simulink model "TestStructure"  (R2023b)
settings: Solver=FixedStepDiscrete  StartTime=0.0  StopTime=inf  FixedStep=SampleTime  RelTol=1e-3
InitFcn:
  | SampleTime = 0.001;
  | ButtonValue=0;
  | load("BusConfig.mat");
undefined symbols (not defined in the file): DiscIntNeverNeededParam
libraries: slrealtimeethercatlib x219, dspfdesign x28, dspstat3 x23, simulink x21, slpidlib x10, dspswit3 x8, commfilt2 x2, dspsigops x1
(part 3 of 8)

== system TestStructure/Bus/Subsystem5/Enabled Subsystem ==
  In1 : Inport
  In2 : Inport  Port=2
  Enable : EnablePort
  Set Device State : slrealtimeethercatlib/Set Device State  device_id=0  slave_name=Drive 2 (Elmo Drive )  sample_time=-1  slave_addr=1002  selected_slave=Term 1 (EK1100)  slave_found=1
  Out1 : Outport
  Out2 : Outport  Port=2
  wires:
  In1/1 -> Set Device State/1
  Set Device State/2 -> Out2/1
  In2/1 -> Set Device State/2
  Set Device State/1 -> Out1/1

== system TestStructure/Bus/Subsystem5/Enabled Subsystem1 ==
  In3 : Inport
  Enable : EnablePort
  EtherCAT Async SDO Upload : slrealtimeethercatlib/EtherCAT Async SDO Upload  index=0x6075  subIndex=0  sig_type=uint32  sig_dim=1  device_id=0  slave_name=Drive 2 (Elmo Drive )  sample_time=-1  slave_addr=1002  selected_slave=Term 1 (EK1100)  timeout=3000  slave_found=1  complete=0
  Out3 : Outport
  Out4 : Outport  Port=2
  Out5 : Outport  Port=3
  wires:
  EtherCAT Async SDO Upload/3 -> Out5/1
  In3/1 -> EtherCAT Async SDO Upload/1
  EtherCAT Async SDO Upload/2 -> Out4/1
  EtherCAT Async SDO Upload/1 -> Out3/1

== system TestStructure/Bus/Subsystem5/Enabled Subsystem2 ==
  In4 : Inport
  In5 : Inport  Port=2
  Enable : EnablePort
  EtherCAT Async SDO Download : slrealtimeethercatlib/EtherCAT Async SDO Download  index=0x6080  subIndex=0  sig_type=int32  sig_dim=1  device_id=0  slave_name=Drive 2 (Elmo Drive )  sample_time=-1  slave_addr=1002  selected_slave=Term 1 (EK1100)  timeout=3000  slave_found=1  complete=0
  Out6 : Outport
  Out7 : Outport  Port=2
  wires:
  EtherCAT Async SDO Download/2 -> Out7/1
  In4/1 -> EtherCAT Async SDO Download/1
  In5/1 -> EtherCAT Async SDO Download/2
  EtherCAT Async SDO Download/1 -> Out6/1

== system TestStructure/Bus/Subsystem5/Enabled Subsystem3 ==
  In6 : Inport
  In7 : Inport  Port=2
  Enable : EnablePort
  EtherCAT Async SDO Download1 : slrealtimeethercatlib/EtherCAT Async SDO Download  index=0x6060  subIndex=0  sig_type=int8  sig_dim=1  device_id=0  slave_name=Drive 2 (Elmo Drive )  sample_time=-1  slave_addr=1002  selected_slave=Term 1 (EK1100)  timeout=2000  slave_found=1  complete=0
  Out8 : Outport
  Out9 : Outport  Port=2
  wires:
  In6/1 -> EtherCAT Async SDO Download1/1
  EtherCAT Async SDO Download1/1 -> Out8/1
  In7/1 -> EtherCAT Async SDO Download1/2
  EtherCAT Async SDO Download1/2 -> Out9/1

== system TestStructure/Bus/Subsystem5/Enabled Subsystem4 ==
  In8 : Inport
  In9 : Inport  Port=2
  Enable : EnablePort
  Set Device State1 : slrealtimeethercatlib/Set Device State  device_id=0  slave_name=Drive 2 (Elmo Drive )  sample_time=-1  slave_addr=1002  selected_slave=Term 1 (EK1100)  slave_found=1
  Out10 : Outport
  Out11 : Outport  Port=2
  wires:
  Set Device State1/1 -> Out10/1
  In8/1 -> Set Device State1/1
  In9/1 -> Set Device State1/2
  Set Device State1/2 -> Out11/1

== system TestStructure/Bus/Subsystem5/Enabled Subsystem5 ==
  Enable : EnablePort
  Get Device State : slrealtimeethercatlib/Get Device State  device_id=0  slave_name=Drive 2 (Elmo Drive )  sample_time=0.001  slave_addr=1002  selected_slave=Term 1 (EK1100)  timeout=500  slave_found=1
  Out12 : Outport
  wires:
  Get Device State/1 -> Out12/1

== system TestStructure/Bus/Subsystem5/Enabled Subsystem6 ==
  In10 : Inport
  Enable : EnablePort
  EtherCAT PDO Receive1 : slrealtimeethercatlib/EtherCAT PDO Receive  Priority=2  sig_name=Drive 2 (Elmo Drive ).Inputs.Status word  sig_offset=12544  sig_type=uint16  type_size=16  sig_dim=1  device_id=0  sample_time=0.001000
  EtherCAT PDO Transmit1 : slrealtimeethercatlib/EtherCAT PDO Transmit  Priority=3  sig_name=Drive 2 (Elmo Drive ).Outputs.Control word  sig_offset=12512  sig_type=uint16  type_size=16  sig_dim=1  device_id=0  sample_time=0.001000
  Out13 : Outport
  wires:
  EtherCAT PDO Receive1/1 -> Out13/1
  In10/1 -> EtherCAT PDO Transmit1/1

== system TestStructure/Bus/Subsystem5/Enabled Subsystem7 ==
  Enable : EnablePort
  EtherCAT PDO Receive2 : slrealtimeethercatlib/EtherCAT PDO Receive  Priority=2  sig_name=Drive 2 (Elmo Drive ).Inputs.Position actual value  sig_offset=12496  sig_type=int32  type_size=32  sig_dim=1  device_id=0  sample_time=0.001000
  Out1 : Outport
  wires:
  EtherCAT PDO Receive2/1 -> Out1/1

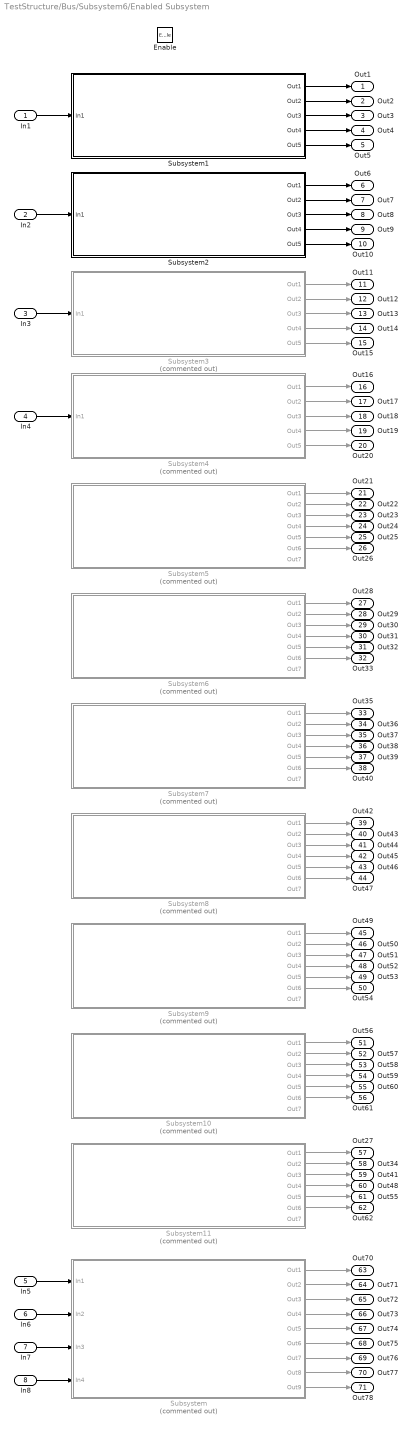
== system TestStructure/Bus/Subsystem6/Enabled Subsystem ==
  In1 : Inport
  In2 : Inport  Port=2
  In3 : Inport  Port=3
  In4 : Inport  Port=4
  In5 : Inport  Port=5
  In6 : Inport  Port=6
  In7 : Inport  Port=7
  In8 : Inport  Port=8
  Enable : EnablePort
  Subsystem : Subsystem  Commented=on
  Subsystem1 : Subsystem
  Subsystem10 : Subsystem  Commented=on
  Subsystem11 : Subsystem  Commented=on
  Subsystem2 : Subsystem
  Subsystem3 : Subsystem  Commented=on
  Subsystem4 : Subsystem  Commented=on
  Subsystem5 : Subsystem  Commented=on
  Subsystem6 : Subsystem  Commented=on
  Subsystem7 : Subsystem  Commented=on
  Subsystem8 : Subsystem  Commented=on
  Subsystem9 : Subsystem  Commented=on
  Out1 : Outport
  Out2 : Outport  Port=2
  Out3 : Outport  Port=3
  Out4 : Outport  Port=4
  Out5 : Outport  Port=5
  Out6 : Outport  Port=6
  Out7 : Outport  Port=7
  Out8 : Outport  Port=8
  Out9 : Outport  Port=9
  Out10 : Outport  Port=10
  Out11 : Outport  Port=11
  Out12 : Outport  Port=12
  Out13 : Outport  Port=13
  Out14 : Outport  Port=14
  Out15 : Outport  Port=15
  Out16 : Outport  Port=16
  Out17 : Outport  Port=17
  Out18 : Outport  Port=18
  Out19 : Outport  Port=19
  Out20 : Outport  Port=20
  Out21 : Outport  Port=21
  Out22 : Outport  Port=22
  Out23 : Outport  Port=23
  Out24 : Outport  Port=24
  Out25 : Outport  Port=25
  Out26 : Outport  Port=26
  Out28 : Outport  Port=27
  Out29 : Outport  Port=28
  Out30 : Outport  Port=29
  Out31 : Outport  Port=30
  Out32 : Outport  Port=31
  Out33 : Outport  Port=32
  Out35 : Outport  Port=33
  Out36 : Outport  Port=34
  Out37 : Outport  Port=35
  Out38 : Outport  Port=36
  Out39 : Outport  Port=37
  Out40 : Outport  Port=38
  Out42 : Outport  Port=39
  Out43 : Outport  Port=40
  Out44 : Outport  Port=41
  Out45 : Outport  Port=42
  Out46 : Outport  Port=43
  Out47 : Outport  Port=44
  Out49 : Outport  Port=45
  Out50 : Outport  Port=46
  Out51 : Outport  Port=47
  Out52 : Outport  Port=48
  Out53 : Outport  Port=49
  Out54 : Outport  Port=50
  Out56 : Outport  Port=51
  Out57 : Outport  Port=52
  Out58 : Outport  Port=53
  Out59 : Outport  Port=54
  Out60 : Outport  Port=55
  Out61 : Outport  Port=56
  Out27 : Outport  Port=57
  Out34 : Outport  Port=58
  Out41 : Outport  Port=59
  Out48 : Outport  Port=60
  Out55 : Outport  Port=61
  Out62 : Outport  Port=62
  Out70 : Outport  Port=63
  Out71 : Outport  Port=64
  Out72 : Outport  Port=65
  Out73 : Outport  Port=66
  Out74 : Outport  Port=67
  Out75 : Outport  Port=68
  Out76 : Outport  Port=69
  Out77 : Outport  Port=70
  Out78 : Outport  Port=71
  wires:
  In1/1 -> Subsystem1/1(In1)
  In2/1 -> Subsystem2/1(In1)
  In3/1 -> Subsystem3/1(In1)
  In4/1 -> Subsystem4/1(In1)
  Subsystem1/1(Out1) -> Out1/1
  Subsystem1/2(Out2) -> Out2/1
  Subsystem1/3(Out3) -> Out3/1
  Subsystem1/4(Out4) -> Out4/1
  Subsystem1/5(Out5) -> Out5/1
  Subsystem2/1(Out1) -> Out6/1
  Subsystem2/2(Out2) -> Out7/1
  Subsystem2/3(Out3) -> Out8/1
  Subsystem2/4(Out4) -> Out9/1
  Subsystem2/5(Out5) -> Out10/1
  Subsystem3/1(Out1) -> Out11/1
  Subsystem3/2(Out2) -> Out12/1
  Subsystem3/3(Out3) -> Out13/1
  Subsystem3/4(Out4) -> Out14/1
  Subsystem3/5(Out5) -> Out15/1
  Subsystem4/1(Out1) -> Out16/1
  Subsystem4/2(Out2) -> Out17/1
  Subsystem4/3(Out3) -> Out18/1
  Subsystem4/4(Out4) -> Out19/1
  Subsystem4/5(Out5) -> Out20/1
  Subsystem5/1(Out1) -> Out21/1
  Subsystem5/2(Out2) -> Out22/1
  Subsystem5/3(Out3) -> Out23/1
  Subsystem5/4(Out4) -> Out24/1
  Subsystem5/5(Out5) -> Out25/1
  Subsystem5/6(Out6) -> Out26/1
  Subsystem6/1(Out1) -> Out28/1
  Subsystem6/2(Out2) -> Out29/1
  Subsystem6/3(Out3) -> Out30/1
  Subsystem6/4(Out4) -> Out31/1
  Subsystem6/5(Out5) -> Out32/1
  Subsystem6/6(Out6) -> Out33/1
  Subsystem7/1(Out1) -> Out35/1
  Subsystem7/2(Out2) -> Out36/1
  Subsystem7/3(Out3) -> Out37/1
  Subsystem7/4(Out4) -> Out38/1
  Subsystem7/5(Out5) -> Out39/1
  Subsystem7/6(Out6) -> Out40/1
  Subsystem8/1(Out1) -> Out42/1
  Subsystem8/2(Out2) -> Out43/1
  Subsystem8/3(Out3) -> Out44/1
  Subsystem8/4(Out4) -> Out45/1
  Subsystem8/5(Out5) -> Out46/1
  Subsystem8/6(Out6) -> Out47/1
  Subsystem9/1(Out1) -> Out49/1
  Subsystem9/2(Out2) -> Out50/1
  Subsystem9/3(Out3) -> Out51/1
  Subsystem9/4(Out4) -> Out52/1
  Subsystem9/5(Out5) -> Out53/1
  Subsystem9/6(Out6) -> Out54/1
  Subsystem10/1(Out1) -> Out56/1
  Subsystem10/2(Out2) -> Out57/1
  Subsystem10/3(Out3) -> Out58/1
  Subsystem10/4(Out4) -> Out59/1
  Subsystem10/5(Out5) -> Out60/1
  Subsystem10/6(Out6) -> Out61/1
  In5/1 -> Subsystem/1(In1)
  In6/1 -> Subsystem/2(In2)
  In7/1 -> Subsystem/3(In3)
  In8/1 -> Subsystem/4(In4)
  Subsystem/1(Out1) -> Out70/1
  Subsystem/2(Out2) -> Out71/1
  Subsystem/3(Out3) -> Out72/1
  Subsystem/4(Out4) -> Out73/1
  Subsystem/5(Out5) -> Out74/1
  Subsystem/6(Out6) -> Out75/1
  Subsystem/7(Out7) -> Out76/1
  Subsystem/8(Out8) -> Out77/1
  Subsystem/9(Out9) -> Out78/1
  Subsystem11/1(Out1) -> Out27/1
  Subsystem11/2(Out2) -> Out34/1
  Subsystem11/3(Out3) -> Out41/1
  Subsystem11/4(Out4) -> Out48/1
  Subsystem11/5(Out5) -> Out55/1
  Subsystem11/6(Out6) -> Out62/1

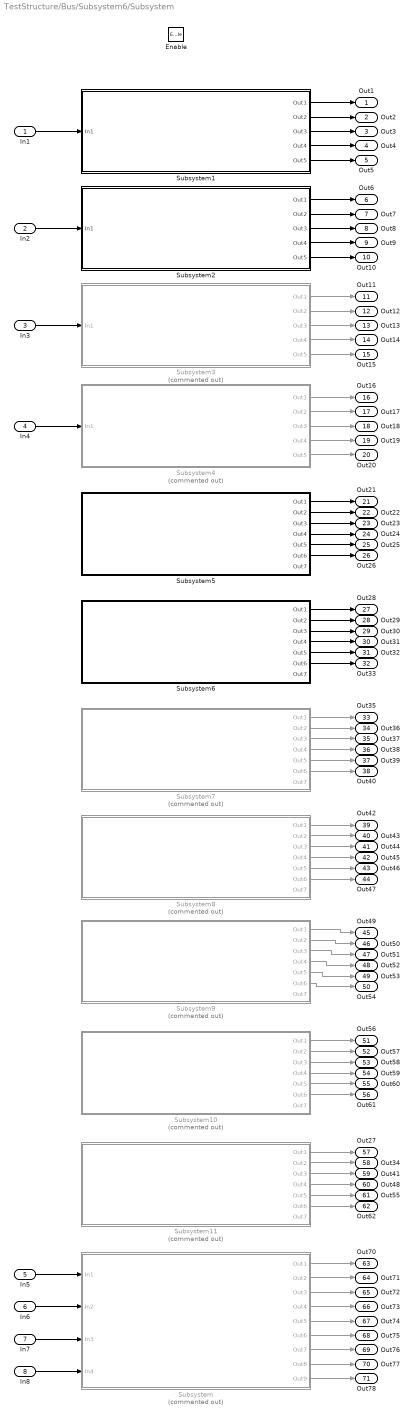
== system TestStructure/Bus/Subsystem6/Subsystem ==
  In1 : Inport
  In2 : Inport  Port=2
  In3 : Inport  Port=3
  In4 : Inport  Port=4
  In5 : Inport  Port=5
  In6 : Inport  Port=6
  In7 : Inport  Port=7
  In8 : Inport  Port=8
  Enable : EnablePort
  Subsystem : Subsystem  Commented=on
  Subsystem1 : Subsystem
  Subsystem10 : Subsystem  Commented=on
  Subsystem11 : Subsystem  Commented=on
  Subsystem2 : Subsystem
  Subsystem3 : Subsystem  Commented=on
  Subsystem4 : Subsystem  Commented=on
  Subsystem5 : Subsystem
  Subsystem6 : Subsystem
  Subsystem7 : Subsystem  Commented=on
  Subsystem8 : Subsystem  Commented=on
  Subsystem9 : Subsystem  Commented=on
  Out1 : Outport
  Out2 : Outport  Port=2
  Out3 : Outport  Port=3
  Out4 : Outport  Port=4
  Out5 : Outport  Port=5
  Out6 : Outport  Port=6
  Out7 : Outport  Port=7
  Out8 : Outport  Port=8
  Out9 : Outport  Port=9
  Out10 : Outport  Port=10
  Out11 : Outport  Port=11
  Out12 : Outport  Port=12
  Out13 : Outport  Port=13
  Out14 : Outport  Port=14
  Out15 : Outport  Port=15
  Out16 : Outport  Port=16
  Out17 : Outport  Port=17
  Out18 : Outport  Port=18
  Out19 : Outport  Port=19
  Out20 : Outport  Port=20
  Out21 : Outport  Port=21
  Out22 : Outport  Port=22
  Out23 : Outport  Port=23
  Out24 : Outport  Port=24
  Out25 : Outport  Port=25
  Out26 : Outport  Port=26
  Out28 : Outport  Port=27
  Out29 : Outport  Port=28
  Out30 : Outport  Port=29
  Out31 : Outport  Port=30
  Out32 : Outport  Port=31
  Out33 : Outport  Port=32
  Out35 : Outport  Port=33
  Out36 : Outport  Port=34
  Out37 : Outport  Port=35
  Out38 : Outport  Port=36
  Out39 : Outport  Port=37
  Out40 : Outport  Port=38
  Out42 : Outport  Port=39
  Out43 : Outport  Port=40
  Out44 : Outport  Port=41
  Out45 : Outport  Port=42
  Out46 : Outport  Port=43
  Out47 : Outport  Port=44
  Out49 : Outport  Port=45
  Out50 : Outport  Port=46
  Out51 : Outport  Port=47
  Out52 : Outport  Port=48
  Out53 : Outport  Port=49
  Out54 : Outport  Port=50
  Out56 : Outport  Port=51
  Out57 : Outport  Port=52
  Out58 : Outport  Port=53
  Out59 : Outport  Port=54
  Out60 : Outport  Port=55
  Out61 : Outport  Port=56
  Out27 : Outport  Port=57
  Out34 : Outport  Port=58
  Out41 : Outport  Port=59
  Out48 : Outport  Port=60
  Out55 : Outport  Port=61
  Out62 : Outport  Port=62
  Out70 : Outport  Port=63
  Out71 : Outport  Port=64
  Out72 : Outport  Port=65
  Out73 : Outport  Port=66
  Out74 : Outport  Port=67
  Out75 : Outport  Port=68
  Out76 : Outport  Port=69
  Out77 : Outport  Port=70
  Out78 : Outport  Port=71
  wires:
  Subsystem/7(Out7) -> Out76/1
  Subsystem5/5(Out5) -> Out25/1
  Subsystem/8(Out8) -> Out77/1
  Subsystem/9(Out9) -> Out78/1
  Subsystem5/1(Out1) -> Out21/1
  Subsystem7/4(Out4) -> Out38/1
  Subsystem/6(Out6) -> Out75/1
  Subsystem/5(Out5) -> Out74/1
  Subsystem4/4(Out4) -> Out19/1
  Subsystem1/1(Out1) -> Out1/1
  Subsystem/3(Out3) -> Out72/1
  Subsystem8/6(Out6) -> Out47/1
  Subsystem/4(Out4) -> Out73/1
  Subsystem8/5(Out5) -> Out46/1
  Subsystem6/6(Out6) -> Out33/1
  Subsystem5/3(Out3) -> Out23/1
  Subsystem3/5(Out5) -> Out15/1
  Subsystem4/5(Out5) -> Out20/1
  Subsystem3/3(Out3) -> Out13/1
  Subsystem2/5(Out5) -> Out10/1
  Subsystem4/1(Out1) -> Out16/1
  Subsystem8/1(Out1) -> Out42/1
  Subsystem8/4(Out4) -> Out45/1
  Subsystem4/3(Out3) -> Out18/1
  Subsystem10/4(Out4) -> Out59/1
  Subsystem8/2(Out2) -> Out43/1
  Subsystem/2(Out2) -> Out71/1
  Subsystem10/2(Out2) -> Out57/1
  Subsystem9/6(Out6) -> Out54/1
  Subsystem4/2(Out2) -> Out17/1
  Subsystem7/6(Out6) -> Out40/1
  Subsystem9/2(Out2) -> Out50/1
  Subsystem7/2(Out2) -> Out36/1
  Subsystem7/3(Out3) -> Out37/1
  Subsystem3/4(Out4) -> Out14/1
  Subsystem5/2(Out2) -> Out22/1
  Subsystem10/6(Out6) -> Out61/1
  Subsystem6/3(Out3) -> Out30/1
  Subsystem2/3(Out3) -> Out8/1
  Subsystem/1(Out1) -> Out70/1
  Subsystem2/1(Out1) -> Out6/1
  Subsystem3/1(Out1) -> Out11/1
  Subsystem5/6(Out6) -> Out26/1
  Subsystem7/5(Out5) -> Out39/1
  Subsystem1/3(Out3) -> Out3/1
  Subsystem3/2(Out2) -> Out12/1
  Subsystem9/3(Out3) -> Out51/1
  Subsystem10/1(Out1) -> Out56/1
  Subsystem6/2(Out2) -> Out29/1
  Subsystem2/2(Out2) -> Out7/1
  Subsystem1/5(Out5) -> Out5/1
  Subsystem9/4(Out4) -> Out52/1
  Subsystem1/4(Out4) -> Out4/1
  Subsystem6/4(Out4) -> Out31/1
  Subsystem5/4(Out4) -> Out24/1
  Subsystem10/5(Out5) -> Out60/1
  Subsystem1/2(Out2) -> Out2/1
  Subsystem2/4(Out4) -> Out9/1
  Subsystem9/5(Out5) -> Out53/1
  Subsystem7/1(Out1) -> Out35/1
  Subsystem6/1(Out1) -> Out28/1
  Subsystem8/3(Out3) -> Out44/1
  Subsystem9/1(Out1) -> Out49/1
  Subsystem10/3(Out3) -> Out58/1
  Subsystem6/5(Out5) -> Out32/1
  In3/1 -> Subsystem3/1(In1)
  In5/1 -> Subsystem/1(In1)
  In2/1 -> Subsystem2/1(In1)
  In1/1 -> Subsystem1/1(In1)
  In8/1 -> Subsystem/4(In4)
  In7/1 -> Subsystem/3(In3)
  In4/1 -> Subsystem4/1(In1)
  In6/1 -> Subsystem/2(In2)
  Subsystem11/1(Out1) -> Out27/1
  Subsystem11/2(Out2) -> Out34/1
  Subsystem11/3(Out3) -> Out41/1
  Subsystem11/4(Out4) -> Out48/1
  Subsystem11/5(Out5) -> Out55/1
  Subsystem11/6(Out6) -> Out62/1

== system TestStructure/Bus/Subsystem6/Subsystem2 ==
  Enable : EnablePort
  Subsystem7 : Subsystem
  Subsystem8 : Subsystem
  Out35 : Outport
  Out36 : Outport  Port=2
  Out37 : Outport  Port=3
  Out38 : Outport  Port=4
  Out42 : Outport  Port=5
  Out43 : Outport  Port=6
  Out44 : Outport  Port=7
  Out45 : Outport  Port=8
  wires:
  Subsystem7/1(Out1) -> Out35/1
  Subsystem8/3(Out3) -> Out44/1
  Subsystem7/4(Out4) -> Out38/1
  Subsystem7/3(Out3) -> Out37/1
  Subsystem8/2(Out2) -> Out43/1
  Subsystem7/2(Out2) -> Out36/1
  Subsystem8/1(Out1) -> Out42/1
  Subsystem8/4(Out4) -> Out45/1

== system TestStructure/Bus/Subsystem7/Enabled Subsystem ==
  In1 : Inport
  In2 : Inport  Port=2
  Enable : EnablePort
  Set Device State : slrealtimeethercatlib/Set Device State  device_id=0  slave_name=Drive 2 (Elmo Drive )  sample_time=-1  slave_addr=1002  selected_slave=Term 1 (EK1100)  slave_found=1
  Out1 : Outport
  Out2 : Outport  Port=2
  wires:
  In1/1 -> Set Device State/1
  Set Device State/2 -> Out2/1
  In2/1 -> Set Device State/2
  Set Device State/1 -> Out1/1

== system TestStructure/Bus/Subsystem7/Enabled Subsystem1 ==
  In3 : Inport
  Enable : EnablePort
  EtherCAT Async SDO Upload : slrealtimeethercatlib/EtherCAT Async SDO Upload  index=0x6075  subIndex=0  sig_type=uint32  sig_dim=1  device_id=0  slave_name=Drive 2 (Elmo Drive )  sample_time=-1  slave_addr=1002  selected_slave=Term 1 (EK1100)  timeout=3000  slave_found=1  complete=0
  Out3 : Outport
  Out4 : Outport  Port=2
  Out5 : Outport  Port=3
  wires:
  EtherCAT Async SDO Upload/3 -> Out5/1
  In3/1 -> EtherCAT Async SDO Upload/1
  EtherCAT Async SDO Upload/2 -> Out4/1
  EtherCAT Async SDO Upload/1 -> Out3/1

== system TestStructure/Bus/Subsystem7/Enabled Subsystem2 ==
  In4 : Inport
  In5 : Inport  Port=2
  Enable : EnablePort
  EtherCAT Async SDO Download : slrealtimeethercatlib/EtherCAT Async SDO Download  index=0x6080  subIndex=0  sig_type=int32  sig_dim=1  device_id=0  slave_name=Drive 2 (Elmo Drive )  sample_time=-1  slave_addr=1002  selected_slave=Term 1 (EK1100)  timeout=3000  slave_found=1  complete=0
  Out6 : Outport
  Out7 : Outport  Port=2
  wires:
  EtherCAT Async SDO Download/2 -> Out7/1
  In4/1 -> EtherCAT Async SDO Download/1
  In5/1 -> EtherCAT Async SDO Download/2
  EtherCAT Async SDO Download/1 -> Out6/1

== system TestStructure/Bus/Subsystem7/Enabled Subsystem3 ==
  In6 : Inport
  In7 : Inport  Port=2
  Enable : EnablePort
  EtherCAT Async SDO Download1 : slrealtimeethercatlib/EtherCAT Async SDO Download  index=0x6060  subIndex=0  sig_type=int8  sig_dim=1  device_id=0  slave_name=Drive 2 (Elmo Drive )  sample_time=-1  slave_addr=1002  selected_slave=Term 1 (EK1100)  timeout=2000  slave_found=1  complete=0
  Out8 : Outport
  Out9 : Outport  Port=2
  wires:
  In6/1 -> EtherCAT Async SDO Download1/1
  EtherCAT Async SDO Download1/1 -> Out8/1
  In7/1 -> EtherCAT Async SDO Download1/2
  EtherCAT Async SDO Download1/2 -> Out9/1

== system TestStructure/Bus/Subsystem7/Enabled Subsystem4 ==
  In8 : Inport
  In9 : Inport  Port=2
  Enable : EnablePort
  Set Device State1 : slrealtimeethercatlib/Set Device State  device_id=0  slave_name=Drive 2 (Elmo Drive )  sample_time=-1  slave_addr=1002  selected_slave=Term 1 (EK1100)  slave_found=1
  Out10 : Outport
  Out11 : Outport  Port=2
  wires:
  Set Device State1/1 -> Out10/1
  In8/1 -> Set Device State1/1
  In9/1 -> Set Device State1/2
  Set Device State1/2 -> Out11/1

== system TestStructure/Bus/Subsystem7/Enabled Subsystem5 ==
  Enable : EnablePort
  Get Device State : slrealtimeethercatlib/Get Device State  device_id=0  slave_name=Drive 2 (Elmo Drive )  sample_time=0.001  slave_addr=1002  selected_slave=Term 1 (EK1100)  timeout=500  slave_found=1
  Out12 : Outport
  wires:
  Get Device State/1 -> Out12/1

== system TestStructure/Bus/Subsystem7/Enabled Subsystem6 ==
  In10 : Inport
  Enable : EnablePort
  EtherCAT PDO Receive1 : slrealtimeethercatlib/EtherCAT PDO Receive  Priority=2  sig_name=Drive 2 (Elmo Drive ).Inputs.Status word  sig_offset=12544  sig_type=uint16  type_size=16  sig_dim=1  device_id=0  sample_time=0.001000
  EtherCAT PDO Transmit1 : slrealtimeethercatlib/EtherCAT PDO Transmit  Priority=3  sig_name=Drive 2 (Elmo Drive ).Outputs.Control word  sig_offset=12512  sig_type=uint16  type_size=16  sig_dim=1  device_id=0  sample_time=0.001000
  Out13 : Outport
  wires:
  EtherCAT PDO Receive1/1 -> Out13/1
  In10/1 -> EtherCAT PDO Transmit1/1

== system TestStructure/Bus/Subsystem7/Enabled Subsystem7 ==
  Enable : EnablePort
  EtherCAT PDO Receive2 : slrealtimeethercatlib/EtherCAT PDO Receive  Priority=2  sig_name=Drive 2 (Elmo Drive ).Inputs.Position actual value  sig_offset=12496  sig_type=int32  type_size=32  sig_dim=1  device_id=0  sample_time=0.001000
  Out1 : Outport
  wires:
  EtherCAT PDO Receive2/1 -> Out1/1

== system TestStructure/InterForceControlTask/AO/Filter ==
  In : Inport
  Highpass Filter : dspfdesign/Highpass Filter  FilterType=IIR  DesignForMinimumOrder=on  FilterOrder=50  StopbandFrequency=0.015  PassbandFrequency=0.3  StopbandAttenuation=80  PassbandRipple=0.1  SampleRateMode=Specify on dialog  SampleRate=1000  SimulateUsing=Interpreted execution  roundingMode=Floor  coeffsDataTypeStr=fixdt(1,16)
  Highpass Filter1 : dspfdesign/Highpass Filter  FilterType=IIR  DesignForMinimumOrder=on  FilterOrder=50  StopbandFrequency=0.29  PassbandFrequency=0.3  StopbandAttenuation=60  PassbandRipple=1  SampleRateMode=Specify on dialog  SampleRate=1000  SimulateUsing=Code generation  roundingMode=Floor  coeffsDataTypeStr=fixdt(1,16)
  Lowpass Filter : dspfdesign/Lowpass Filter  FilterType=IIR  DesignForMinimumOrder=on  FilterOrder=50  PassbandFrequency=2.3  StopbandFrequency=4.3  PassbandRipple=0.1  StopbandAttenuation=80  SampleRateMode=Specify on dialog  SampleRate=1000  SimulateUsing=Interpreted execution  roundingMode=Floor  coeffsDataTypeStr=fixdt(1,16)
  Lowpass Filter1 : dspfdesign/Lowpass Filter  FilterType=IIR  DesignForMinimumOrder=on  FilterOrder=50  PassbandFrequency=6  StopbandFrequency=8  PassbandRipple=1  StopbandAttenuation=60  SampleRateMode=Specify on dialog  SampleRate=1000  SimulateUsing=Code generation  roundingMode=Floor  coeffsDataTypeStr=fixdt(1,16)
  Out : Outport
  wires:
  Highpass Filter1/1 -> Lowpass Filter1/1
  In/1 -> Highpass Filter1/1
  Lowpass Filter1/1 -> Out/1
  Highpass Filter/1 -> Lowpass Filter/1

== system TestStructure/InterForceControlTask/AO/PhaseCorrection ==
  note: Subsystem
  Peaks : Inport
  T_base_default : Inport  Port=2
  Clock : Clock
  Constant3 : Constant
  Discrete-Time Integrator : DiscreteIntegrator  ExternalReset=rising  SampleTime=-1  ICPrevOutput=DiscIntNeverNeededParam  ICPrevScaledInput=DiscIntNeverNeededParam
  If : If  IfExpression=u1 == 1
  If Action Subsystem : Subsystem  TreatAsAtomicUnit=on
  If Action Subsystem1 : Subsystem  TreatAsAtomicUnit=on
  MATLAB Function : MATLAB Function  TreatAsAtomicUnit=on
  MATLAB Function1 : MATLAB Function  TreatAsAtomicUnit=on
  MATLAB Function2 : MATLAB Function  TreatAsAtomicUnit=on
  Merge : Merge
  Omega : Outport  OutputWhenDisabled=reset  InitialOutput=[0]
  Phi_Corrected : Outport  Port=2  OutputWhenDisabled=reset  InitialOutput=[0]
  wires:
  Clock/1 -> MATLAB Function1/2(t)
  Peaks/1 -> MATLAB Function2/1(valid_peak), If/1, MATLAB Function1/1(raw_peak)
  If/1 -> If Action Subsystem/Action
  Discrete-Time Integrator/1 -> MATLAB Function/1(t_t_start)
  If/2 -> If Action Subsystem1/Action
  Merge/1 -> Discrete-Time Integrator/2, MATLAB Function/2(u)
  Constant3/1 -> Discrete-Time Integrator/1
  If Action Subsystem1/1(Out1) -> Merge/2
  If Action Subsystem/1(Out1) -> Merge/1
  MATLAB Function/1(Omega) -> Omega/1
  MATLAB Function/2(phi) -> Phi_Corrected/1
  T_base_default/1 -> MATLAB Function/3(T_base_default)

== system TestStructure/InterForceControlTask/AO/Select ==
  P : Inport
  Phi : Inport  Port=2
  q : Inport  Port=3
  Abs : Abs  SaturateOnIntegerOverflow=off
  Add : Sum
  Bias1 : Bias  SaturateOnIntegerOverflow=off
  Bias2 : Bias  Bias=-0.001  SaturateOnIntegerOverflow=off
  Constant1 : Constant
  Data Type Conversion : DataTypeConversion  OutDataTypeStr=double  SaturateOnIntegerOverflow=off  RndMeth=Floor
  Edge Detector : dspswit3/Edge Detector
  Gain1 : Gain  Gain=0.6
  Gain2 : Gain  OutDataTypeStr=Inherit: Same as input  ParamDataTypeStr=Inherit: Same as input
  Gain3 : Gain  Gain=0.4
  If Action Subsystem : Subsystem  TreatAsAtomicUnit=on
  If Action Subsystem1 : Subsystem  TreatAsAtomicUnit=on
  If1 : If  NumInputs=3  IfExpression=(u1 >= 10.5)|(u2 <= u3)
  MATLAB Function1 : MATLAB Function  TreatAsAtomicUnit=on
  MO_AOActivityMovment : Sum
  MO_AOActivityThreadhold : Constant  Value=0
  Merge : Merge
  Merge1 : Merge
  Merge2 : Merge
  Moving Average : dspstat3/Moving Average  Method=Sliding window  ForgettingFactorPort=off  SpecifyWindowLength=on  WindowLength=2000  OverlapLength=1999  AllowArbitraryInputLength=off  ForgettingFactor=0.9  SimulateUsing=Code generation
  Moving Average1 : dspstat3/Moving Average  Method=Sliding window  ForgettingFactorPort=off  SpecifyWindowLength=on  WindowLength=2000  OverlapLength=1999  AllowArbitraryInputLength=off  ForgettingFactor=0.9  SimulateUsing=Code generation
  Saturation : Saturate  UpperLimit=inf  LowerLimit=0
  Phi_Out : Outport
  Phase0Event : Outport  Port=2
  PhaseEn : Outport  Port=3
  wires:
  Merge2/1 -> PhaseEn/1
  If Action Subsystem/3(En) -> Merge2/2
  If Action Subsystem1/3(Out3) -> Merge2/1
  Constant1/1 -> If1/1
  Bias1/1 -> If Action Subsystem/2(Phase0)
  If Action Subsystem/2(Phase0Event) -> Merge1/2
  If Action Subsystem1/2(Out2) -> Merge1/1
  If Action Subsystem/1(Phi_Out) -> Merge/2
  MO_AOActivityMovment/1 -> If1/2
  Data Type Conversion/1 -> Gain2/1
  Gain3/1 -> MO_AOActivityMovment/1
  Moving Average1/1 -> MO_AOActivityMovment/2
  q/1 -> MATLAB Function1/1(u)
  MATLAB Function1/1(y) -> Abs/1
  Abs/1 -> Moving Average1/1, Gain3/1
  Merge1/1 -> Phase0Event/1
  Merge/1 -> Phi_Out/1
  If1/2 -> If Action Subsystem/Action
  Add/1 -> ?
  If1/1 -> If Action Subsystem1/Action
  Gain2/1 -> Bias1/1
  Moving Average/1 -> Add/2
  Saturation/1 -> Edge Detector/1
  Edge Detector/1 -> Data Type Conversion/1
  Phi/1 -> If Action Subsystem/1(Phi), Bias2/1
  Bias2/1 -> Saturation/1
  P/1 -> Moving Average/1, Gain1/1
  Gain1/1 -> Add/1
  If Action Subsystem1/1(Out1) -> Merge/1
  MO_AOActivityThreadhold/1 -> If1/3

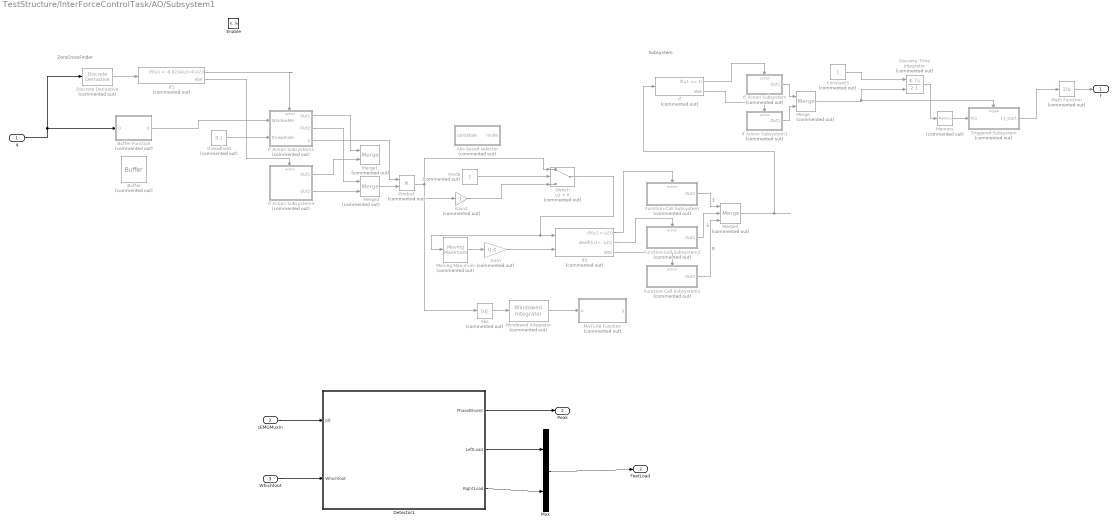
== system TestStructure/InterForceControlTask/AO/Subsystem1 ==
  note: ZeroCrossFinder
  note: Subsystem
  q : Inport
  sEMGMuxIn : Inport  Port=2
  Whichfoot : Inport  Port=3
  Enable : EnablePort  StatesWhenEnabling=reset
  Abs : Abs  Commented=on  SaturateOnIntegerOverflow=off
  Abs-based selector : Subsystem  Commented=on
  Buffer : Buffer  Commented=on  N=30  V=29  OutputFrames=off
  Buffer Function : MATLAB Function  Commented=on  TreatAsAtomicUnit=on
  Constant3 : Constant  Commented=on
  Detector1 : Subsystem
  Discrete Derivative : simulink/Discrete/Discrete Derivative  Commented=on  gainval=1.0  ICPrevScaledInput=0.0  OutMin=[]  OutMax=[]  OutDataType=fixdt(1, 16)  OutScaling=2^-10  DoSatur=off
  Discrete-Time Integrator : DiscreteIntegrator  Commented=on  ExternalReset=rising  SampleTime=-1  ICPrevOutput=DiscIntNeverNeededParam  ICPrevScaledInput=DiscIntNeverNeededParam
  Function-Call Subsystem : Subsystem  Commented=on  TreatAsAtomicUnit=on
  Function-Call Subsystem1 : Subsystem  Commented=on  TreatAsAtomicUnit=on
  Function-Call Subsystem2 : Subsystem  Commented=on  TreatAsAtomicUnit=on
  Gain : Gain  Commented=on  Gain=0.4
  Gain2 : Gain  Commented=on  Gain=-1
  If : If  Commented=on  IfExpression=u1 == 1
  If Action Subsystem : Subsystem  Commented=on  TreatAsAtomicUnit=on
  If Action Subsystem1 : Subsystem  Commented=on  TreatAsAtomicUnit=on
  If Action Subsystem2 : Subsystem  Commented=on  TreatAsAtomicUnit=on
  If Action Subsystem3 : Subsystem  Commented=on  TreatAsAtomicUnit=on
  If1 : If  Commented=on  IfExpression=(u1 > -0.02)&(u1<0.02)
  If2 : If  Commented=on  NumInputs=2  IfExpression=(u1 > u2)  ElseIfExpressions=(u1< -u2)
  MATLAB Function : MATLAB Function  Commented=on  TreatAsAtomicUnit=on
  Math Function : Math  Commented=on  Operator=reciprocal
  Memory : Memory  Commented=on
  Merge : Merge  Commented=on
  Merge1 : Merge  Commented=on
  Merge2 : Merge  Commented=on
  Merge3 : Merge  Commented=on  Inputs=3
  Moving Maximum : dspstat3/Moving Maximum  Commented=on  SpecifyWindowLength=on  WindowLength=2000  SimulateUsing=Code generation
  Mux : Mux  Inputs=2
  Product : Product  Commented=on
  Switch : Switch  Commented=on  Criteria=u2 > Threshold  SaturateOnIntegerOverflow=off  InputSameDT=off
  Triggered Subsystem : Subsystem  Commented=on  TreatAsAtomicUnit=on
  Windowed Integrator : commfilt2/Windowed Integrator  Commented=on  integperiod=600  roundingMode=Floor  overflowMode=off  coeffDataTypeStr=Inherit: Same word length as input  coeffMin=[]  coeffMax=[]  coeffLastDataTypeStr=Inherit: Same word length as input  accumDataTypeStr=Inherit: Same as product output  accumLastDataTypeStr=Inherit: Same as product output  outputDataTypeStr=Inherit: Same as accumulator  outputMin=[]  outputMax=[]  outputLastDataTypeStr=Inherit: Same as accumulator
  mode : Constant  Commented=on
  threadhold : Constant  Commented=on  Value=0.1
  f : Outport
  Peak : Outport  Port=2  OutputWhenDisabled=reset  InitialOutput=[0]
  FeetLoad : Outport  Port=3  OutputWhenDisabled=reset  InitialOutput=[0]
  wires:
  Triggered Subsystem/1(t-t_start) -> Math Function/1
  Math Function/1 -> f/1
  Memory/1 -> Triggered Subsystem/1(In1)
  If Action Subsystem/1(Out1) -> Merge/1
  If Action Subsystem1/1(Out1) -> Merge/2
  Constant3/1 -> Discrete-Time Integrator/1
  If/1 -> If Action Subsystem/Action
  Merge/1 -> Discrete-Time Integrator/2, Triggered Subsystem/Trigger
  If/2 -> If Action Subsystem1/Action
  Discrete-Time Integrator/1 -> Memory/1
  q/1 -> Discrete Derivative/1, Buffer Function/1(u)
  If Action Subsystem3/1(Out1) -> Merge1/2
  If Action Subsystem2/1(Out1) -> Merge1/1
  If1/2 -> If Action Subsystem3/Action
  If1/1 -> If Action Subsystem2/Action
  Discrete Derivative/1 -> If1/1
  Buffer Function/1(y) -> If Action Subsystem2/1(WindowMin)
  If Action Subsystem2/2(Out2) -> Merge2/1
  If Action Subsystem3/2(Out2) -> Merge2/2
  Merge2/1 -> Product/2
  If Action Subsystem2/3(y) -> Product/1
  Function-Call Subsystem/1(Out1) -> Merge3/1  "1"
  Function-Call Subsystem1/1(Out1) -> Merge3/3  "0"
  If2/1 -> Function-Call Subsystem/Action
  If2/3 -> Function-Call Subsystem1/Action
  Function-Call Subsystem2/1(Out1) -> Merge3/2  "-1"
  If2/2 -> Function-Call Subsystem2/Action
  Moving Maximum/1 -> Gain/1
  Gain/1 -> If2/2
  Product/1 -> Switch/1, Abs/1, Gain2/1
  Switch/1 -> Moving Maximum/1, If2/1
  Gain2/1 -> Switch/3
  threadhold/1 -> If Action Subsystem2/2(threadhold)
  Abs/1 -> Windowed Integrator/1
  Windowed Integrator/1 -> MATLAB Function/1(u)
  mode/1 -> Switch/2
  Merge3/1 -> If/1
  Detector1/1(Phase0Event) -> Peak/1
  sEMGMuxIn/1 -> Detector1/1(p8)
  Whichfoot/1 -> Detector1/2(Whichfoot)
  Detector1/2(LeftLoad) -> Mux/1
  Detector1/3(RightLoad) -> Mux/2
  Mux/1 -> FeetLoad/1

== system TestStructure/InterForceControlTask/AO1/Filter ==
  In : Inport
  Highpass Filter : dspfdesign/Highpass Filter  FilterType=IIR  DesignForMinimumOrder=on  FilterOrder=50  StopbandFrequency=0.015  PassbandFrequency=0.3  StopbandAttenuation=80  PassbandRipple=0.1  SampleRateMode=Specify on dialog  SampleRate=1000  SimulateUsing=Interpreted execution  roundingMode=Floor  coeffsDataTypeStr=fixdt(1,16)
  Highpass Filter1 : dspfdesign/Highpass Filter  FilterType=IIR  DesignForMinimumOrder=on  FilterOrder=50  StopbandFrequency=0.2  PassbandFrequency=0.3  StopbandAttenuation=60  PassbandRipple=1  SampleRateMode=Specify on dialog  SampleRate=1000  SimulateUsing=Code generation  roundingMode=Floor  coeffsDataTypeStr=fixdt(1,16)
  Lowpass Filter : dspfdesign/Lowpass Filter  FilterType=IIR  DesignForMinimumOrder=on  FilterOrder=50  PassbandFrequency=2.3  StopbandFrequency=4.3  PassbandRipple=0.1  StopbandAttenuation=80  SampleRateMode=Specify on dialog  SampleRate=1000  SimulateUsing=Interpreted execution  roundingMode=Floor  coeffsDataTypeStr=fixdt(1,16)
  Lowpass Filter1 : dspfdesign/Lowpass Filter  FilterType=IIR  DesignForMinimumOrder=on  FilterOrder=50  PassbandFrequency=6  StopbandFrequency=8  PassbandRipple=1  StopbandAttenuation=60  SampleRateMode=Specify on dialog  SampleRate=1000  SimulateUsing=Code generation  roundingMode=Floor  coeffsDataTypeStr=fixdt(1,16)
  Out : Outport
  wires:
  Highpass Filter1/1 -> Lowpass Filter1/1
  In/1 -> Highpass Filter/1
  Lowpass Filter/1 -> Out/1
  Highpass Filter/1 -> Lowpass Filter/1

== system TestStructure/InterForceControlTask/AO1/PhaseCorrection ==
  note: Subsystem
  Peaks : Inport
  Clock : Clock
  Constant3 : Constant
  Discrete-Time Integrator : DiscreteIntegrator  ExternalReset=rising  SampleTime=-1  ICPrevOutput=DiscIntNeverNeededParam  ICPrevScaledInput=DiscIntNeverNeededParam
  If : If  IfExpression=u1 == 1
  If Action Subsystem : Subsystem  TreatAsAtomicUnit=on
  If Action Subsystem1 : Subsystem  TreatAsAtomicUnit=on
  MATLAB Function : MATLAB Function  TreatAsAtomicUnit=on
  MATLAB Function1 : MATLAB Function  TreatAsAtomicUnit=on
  MATLAB Function2 : MATLAB Function  TreatAsAtomicUnit=on
  Merge : Merge
  Omega : Outport  OutputWhenDisabled=reset  InitialOutput=[0]
  Phi_Corrected : Outport  Port=2  OutputWhenDisabled=reset  InitialOutput=[0]
  wires:
  Clock/1 -> MATLAB Function1/2(t)
  MATLAB Function1/1(valid_peak) -> If/1, MATLAB Function2/1(valid_peak)
  Peaks/1 -> MATLAB Function1/1(raw_peak)
  If/1 -> If Action Subsystem/Action
  Discrete-Time Integrator/1 -> MATLAB Function/1(t_t_start)
  If/2 -> If Action Subsystem1/Action
  Merge/1 -> Discrete-Time Integrator/2, MATLAB Function/2(u)
  Constant3/1 -> Discrete-Time Integrator/1
  If Action Subsystem1/1(Out1) -> Merge/2
  If Action Subsystem/1(Out1) -> Merge/1
  MATLAB Function/1(Omega) -> Omega/1
  MATLAB Function/2(phi) -> Phi_Corrected/1

== system TestStructure/InterForceControlTask/AO1/Select ==
  P : Inport
  Phi : Inport  Port=2
  q : Inport  Port=3
  Abs : Abs  SaturateOnIntegerOverflow=off
  Add : Sum
  Add1 : Sum
  Bias1 : Bias  SaturateOnIntegerOverflow=off
  Bias2 : Bias  Bias=-0.001  SaturateOnIntegerOverflow=off
  Constant1 : Constant
  Data Type Conversion : DataTypeConversion  OutDataTypeStr=double  SaturateOnIntegerOverflow=off  RndMeth=Floor
  Edge Detector : dspswit3/Edge Detector
  Gain1 : Gain  Gain=0.6
  Gain2 : Gain  OutDataTypeStr=Inherit: Same as input  ParamDataTypeStr=Inherit: Same as input
  Gain3 : Gain  Gain=0.6
  If : If  NumInputs=2  IfExpression=(u1 >= 10.5)|(u2 <= 1.5)
  If Action Subsystem : Subsystem  TreatAsAtomicUnit=on
  If Action Subsystem1 : Subsystem  TreatAsAtomicUnit=on
  MATLAB Function1 : MATLAB Function  TreatAsAtomicUnit=on
  Merge : Merge
  Merge1 : Merge
  Merge2 : Merge
  Moving Average : dspstat3/Moving Average  Method=Sliding window  ForgettingFactorPort=off  SpecifyWindowLength=on  WindowLength=2000  OverlapLength=1999  AllowArbitraryInputLength=off  ForgettingFactor=0.9  SimulateUsing=Code generation
  Moving Average1 : dspstat3/Moving Average  Method=Sliding window  ForgettingFactorPort=off  SpecifyWindowLength=on  WindowLength=2000  OverlapLength=1999  AllowArbitraryInputLength=off  ForgettingFactor=0.9  SimulateUsing=Code generation
  Saturation : Saturate  UpperLimit=inf  LowerLimit=0
  Phi_Out : Outport
  Phase0Event : Outport  Port=2
  PhaseEn : Outport  Port=3
  wires:
  Merge2/1 -> PhaseEn/1
  If Action Subsystem/3(En) -> Merge2/2
  If Action Subsystem1/3(Out3) -> Merge2/1
  Constant1/1 -> If/1
  Bias1/1 -> If Action Subsystem/2(Phase0)
  If Action Subsystem/2(Phase0Event) -> Merge1/2
  If Action Subsystem1/2(Out2) -> Merge1/1
  If Action Subsystem/1(Phi_Out) -> Merge/2
  Add1/1 -> If/2
  Data Type Conversion/1 -> Gain2/1
  Gain3/1 -> Add1/1
  Moving Average1/1 -> Add1/2
  q/1 -> MATLAB Function1/1(u)
  MATLAB Function1/1(y) -> Abs/1
  Abs/1 -> Moving Average1/1, Gain3/1
  Merge1/1 -> Phase0Event/1
  Merge/1 -> Phi_Out/1
  If/2 -> If Action Subsystem/Action
  Add/1 -> ?
  If/1 -> If Action Subsystem1/Action
  Gain2/1 -> Bias1/1
  Moving Average/1 -> Add/2
  Saturation/1 -> Edge Detector/1
  Edge Detector/1 -> Data Type Conversion/1
  Phi/1 -> If Action Subsystem/1(Phi), Bias2/1
  Bias2/1 -> Saturation/1
  P/1 -> Moving Average/1, Gain1/1
  Gain1/1 -> Add/1
  If Action Subsystem1/1(Out1) -> Merge/1

== system TestStructure/InterForceControlTask/AO1/Subsystem ==
  q : Inport
  f : Inport  Port=2
  Add : Sum  Inputs=++++
  Gain1 : Gain  Gain=1/(2*pi)
  Gain2 : Gain  Gain=1/(2*pi)
  Subsystem : Subsystem
      settings: PortSchema="{\"entries\":[{\"content\":{\"sides\":[{\"content\":{\"connectorIds\":[\"In1\",\"In2\",\"In3\"]},\"type\":\"ConnectorPlacement.EquallySpacedRectSide\",\"uuid\":\"fcadf485-1c54-4f3f-872d-ec2f9b882f19\"},{\"content\":{\"connectorIds\":[\"Out1\",\"Out2\",\"Out3\",\"Out4\"],\"side\":\"RIGHT\"},\"type\":\"ConnectorPlacement.EquallySpacedRectSide\",\"uuid\":\"c1591880-cfe2-422f-a22e-44609bf238b6\"},{\"content\":{\"connectorIds\":[\"In4\"],\"side\":\"TOP\"},\"type\":\"ConnectorPlacement.EquallySpacedRectSide\",\"uuid\":\"5e5eda86-5041-4cab-91db-6a7c0e12be81\"}]},\"type\":\"ConnectorPlacement.EquallySpacedConnector\",\"uuid\":\"19c16159-ed31-430a-9428-452ee8c26aba\"}],\"packageUris\":[\"http://schema.mathworks.com/mf0/Connector/R2020b\"],\"version\":\"1.0\"}"
  Subsystem1 : Subsystem
  Subsystem2 : Subsystem
      settings: PortSchema="{\"entries\":[{\"content\":{\"sides\":[{\"content\":{\"connectorIds\":[\"In1\",\"In2\",\"In3\"]},\"type\":\"ConnectorPlacement.EquallySpacedRectSide\",\"uuid\":\"8ec379b7-ae46-4480-a29c-58696021cca5\"},{\"content\":{\"connectorIds\":[\"Out1\",\"Out2\",\"Out3\"],\"side\":\"RIGHT\"},\"type\":\"ConnectorPlacement.EquallySpacedRectSide\",\"uuid\":\"cda231b2-17f5-4d36-92f5-7ce39ba724b7\"},{\"content\":{\"connectorIds\":[],\"side\":\"TOP\"},\"type\":\"ConnectorPlacement.EquallySpacedRectSide\",\"uuid\":\"4db6421b-b56f-479d-b059-30db4d04c79c\"},{\"content\":{\"connectorIds\":[\"Out4\"],\"side\":\"BOTTOM\"},\"type\":\"ConnectorPlacement.EquallySpacedRectSide\",\"uuid\":\"ff0451e3-8881-4680-9eeb-8c81f572143a\"}]},\"type\":\"ConnectorPlacement.EquallySpacedConnector\",\"uuid\":\"26cfb436-360b-4c37-a6b2-80fa044f0317\"}],\"packageUris\":[\"http://schema.mathworks.com/mf0/Connector/R2020b\"],\"version\":\"1.0\"}"
  Subsystem3 : Subsystem
  Subsystem5 : Subsystem
  x : Outport
  Omega : Outport  Port=2
  Phi : Outport  Port=3
  P : Outport  Port=4
  wires:
  f/1 -> Subsystem/4(f)
  Subsystem/2(Omega) -> Subsystem1/3(Omega), Subsystem3/2(Omega), Subsystem5/3(Omega), Gain1/1
  Subsystem2/4(P) -> P/1
  Subsystem5/1(x) -> Add/4
  Subsystem3/1(x) -> Add/3
  Subsystem2/3(P(t)_Phi) -> Subsystem/3(P(t)_Phi), Subsystem1/2(P(t)_Phi), Subsystem3/3(P(t)_Phi), Subsystem5/2(P(t)_Phi)
  Subsystem1/1(x) -> Add/2
  Subsystem2/2(P(t)_Omega) -> Subsystem/2(P(t)_Omega)
  Subsystem2/1(P(t)_x) -> Subsystem/1(P(t)_x), Subsystem1/1(P(t)_x), Subsystem3/1(P(t)_x), Subsystem5/1(P(t)_x)
  Gain1/1 -> Omega/1
  Subsystem/3(Phi) -> Gain2/1
  Subsystem/1(x) -> Add/1
  Gain2/1 -> Phi/1
  Add/1 -> x/1, Subsystem2/2(X(t))
  q/1 -> Subsystem2/1(T(t))

== system TestStructure/InterForceControlTask/AO1/Subsystem1 ==
  note: Subsystem
  note: ZeroCrossFinder
  q : Inport
  Enable : EnablePort  StatesWhenEnabling=reset
  Constant3 : Constant
  Discrete Derivative : simulink/Discrete/Discrete Derivative  gainval=1.0  ICPrevScaledInput=0.0  OutMin=[]  OutMax=[]  OutDataType=fixdt(1, 16)  OutScaling=2^-10  DoSatur=off
  Discrete-Time Integrator : DiscreteIntegrator  ExternalReset=rising  SampleTime=-1  ICPrevOutput=DiscIntNeverNeededParam  ICPrevScaledInput=DiscIntNeverNeededParam
  If : If  IfExpression=u1 == 1
  If Action Subsystem : Subsystem  TreatAsAtomicUnit=on
  If Action Subsystem1 : Subsystem  TreatAsAtomicUnit=on
  If Action Subsystem2 : Subsystem  TreatAsAtomicUnit=on
  If Action Subsystem3 : Subsystem  TreatAsAtomicUnit=on
  If1 : If  IfExpression=(u1 > -0.005)|(u1<0.005)
  Math Function : Math  Operator=reciprocal
  Memory : Memory
  Merge : Merge
  Merge1 : Merge
  Moving Minimum : dspstat3/Moving Minimum  SpecifyWindowLength=on  WindowLength=3  SimulateUsing=Code generation
  Triggered Subsystem : Subsystem  TreatAsAtomicUnit=on
  f : Outport
  Peak : Outport  Port=2  OutputWhenDisabled=reset  InitialOutput=[0]
  wires:
  Discrete Derivative/1 -> If1/1
  If1/1 -> If Action Subsystem2/Action
  If1/2 -> If Action Subsystem3/Action
  If Action Subsystem2/1(Out1) -> Merge1/1
  If Action Subsystem3/1(Out1) -> Merge1/2
  q/1 -> Discrete Derivative/1, Moving Minimum/1
  Moving Minimum/1 -> If Action Subsystem2/1(WindowMin)
  Discrete-Time Integrator/1 -> Memory/1
  Merge1/1 -> Peak/1, If/1
  If/2 -> If Action Subsystem1/Action
  Merge/1 -> Triggered Subsystem/Trigger, Discrete-Time Integrator/2
  If/1 -> If Action Subsystem/Action
  Constant3/1 -> Discrete-Time Integrator/1
  If Action Subsystem1/1(Out1) -> Merge/2
  If Action Subsystem/1(Out1) -> Merge/1
  Memory/1 -> Triggered Subsystem/1(In1)
  Math Function/1 -> f/1
  Triggered Subsystem/1(t-t_start) -> Math Function/1

== system TestStructure/InterForceControlTask/AO2/Filter ==
  In : Inport
  Highpass Filter : dspfdesign/Highpass Filter  FilterType=IIR  DesignForMinimumOrder=on  FilterOrder=50  StopbandFrequency=0.015  PassbandFrequency=0.3  StopbandAttenuation=80  PassbandRipple=0.1  SampleRateMode=Specify on dialog  SampleRate=1000  SimulateUsing=Interpreted execution  roundingMode=Floor  coeffsDataTypeStr=fixdt(1,16)
  Highpass Filter1 : dspfdesign/Highpass Filter  Commented=on  FilterType=IIR  DesignForMinimumOrder=on  FilterOrder=50  StopbandFrequency=0.2  PassbandFrequency=0.3  StopbandAttenuation=60  PassbandRipple=1  SampleRateMode=Specify on dialog  SampleRate=1000  SimulateUsing=Code generation  roundingMode=Floor  coeffsDataTypeStr=fixdt(1,16)
  Lowpass Filter : dspfdesign/Lowpass Filter  FilterType=IIR  DesignForMinimumOrder=on  FilterOrder=50  PassbandFrequency=2.3  StopbandFrequency=4.3  PassbandRipple=0.1  StopbandAttenuation=80  SampleRateMode=Specify on dialog  SampleRate=1000  SimulateUsing=Interpreted execution  roundingMode=Floor  coeffsDataTypeStr=fixdt(1,16)
  Lowpass Filter1 : dspfdesign/Lowpass Filter  Commented=on  FilterType=IIR  DesignForMinimumOrder=on  FilterOrder=50  PassbandFrequency=6  StopbandFrequency=8  PassbandRipple=1  StopbandAttenuation=60  SampleRateMode=Specify on dialog  SampleRate=1000  SimulateUsing=Code generation  roundingMode=Floor  coeffsDataTypeStr=fixdt(1,16)
  Out : Outport
  wires:
  Highpass Filter1/1 -> Lowpass Filter1/1
  In/1 -> Highpass Filter/1
  Lowpass Filter/1 -> Out/1
  Highpass Filter/1 -> Lowpass Filter/1

== system TestStructure/InterForceControlTask/AO2/PhaseCorrection ==
  Peaks : Inport
  Phi_GP : Inport  Port=2
  Omega : Inport  Port=3
  Reset : Inport  Port=4
  Constant : Constant  Value=0
  Discrete-Time Integrator : DiscreteIntegrator  ExternalReset=falling  InitialConditionSource=external  SampleTime=-1  ICPrevOutput=DiscIntNeverNeededParam  ICPrevScaledInput=DiscIntNeverNeededParam
  Gain : Gain  Gain=-1
  Math Function : Math
  Product : Product  Inputs=4
  Product1 : Product
  Subsystem : Subsystem
  Subsystem1 : Subsystem
  Subsystem2 : Subsystem
  Subsystem3 : Subsystem
  Subsystem4 : Subsystem
  Subsystem5 : Subsystem
  Subtract : Sum  Inputs=+-
  Phi_Corrected : Outport
  wires:
  Subsystem4/1(k_e) -> Product/1
  Constant/1 -> Discrete-Time Integrator/3
  Subsystem5/1(Phi_Corrected) -> Phi_Corrected/1
  Reset/1 -> Subsystem4/1(Reset), Discrete-Time Integrator/2
  Math Function/1 -> Product/4
  Product1/1 -> Math Function/1
  Gain/1 -> Product1/2
  Omega/1 -> Gain/1, Product/3
  Subtract/1 -> Product/2
  Subsystem3/1(Phi_e(t_start)) -> Subtract/2
  Subsystem2/1(P_e(t_start)) -> Subtract/1
  Subsystem1/1(Phi_GP(t_start)) -> Subsystem2/1(Phi_GP(t_start))
  Product/1 -> Discrete-Time Integrator/1
  Discrete-Time Integrator/1 -> Subsystem5/1(Phi_e), Subsystem3/2(Phi_e(t))  "Phi_e"
  Phi_GP/1 -> Subsystem1/2(Phi_GP(t)), Subsystem5/2(Phi_GP)
  Subsystem/1(t-t_start) -> Product1/1
  Peaks/1 -> Subsystem/1(Peaks), Subsystem1/1(Peaks), Subsystem3/1(Peaks)

== system TestStructure/InterForceControlTask/AO2/Select ==
  P : Inport
  Phi : Inport  Port=2
  q : Inport  Port=3
  Abs : Abs  SaturateOnIntegerOverflow=off
  Add : Sum
  Add1 : Sum
  Bias1 : Bias  SaturateOnIntegerOverflow=off
  Bias2 : Bias  Bias=-0.001  SaturateOnIntegerOverflow=off
  Data Type Conversion : DataTypeConversion  OutDataTypeStr=double  SaturateOnIntegerOverflow=off  RndMeth=Floor
  Edge Detector : dspswit3/Edge Detector
  Gain1 : Gain  Gain=0.6
  Gain2 : Gain  OutDataTypeStr=Inherit: Same as input  ParamDataTypeStr=Inherit: Same as input
  Gain3 : Gain  Gain=0.6
  If : If  NumInputs=2  IfExpression=(u1 >= 13.0)|(u2 <= 1)
  If Action Subsystem : Subsystem  TreatAsAtomicUnit=on
  If Action Subsystem1 : Subsystem  TreatAsAtomicUnit=on
  MATLAB Function1 : MATLAB Function  TreatAsAtomicUnit=on
  Merge : Merge
  Merge1 : Merge
  Moving Average : dspstat3/Moving Average  Method=Sliding window  ForgettingFactorPort=off  SpecifyWindowLength=on  WindowLength=2000  OverlapLength=1999  AllowArbitraryInputLength=off  ForgettingFactor=0.9  SimulateUsing=Code generation
  Moving Average1 : dspstat3/Moving Average  Method=Sliding window  ForgettingFactorPort=off  SpecifyWindowLength=on  WindowLength=2000  OverlapLength=1999  AllowArbitraryInputLength=off  ForgettingFactor=0.9  SimulateUsing=Code generation
  Saturation : Saturate  UpperLimit=inf  LowerLimit=0
  Phi_Out : Outport
  Phase0Event : Outport  Port=2
  wires:
  Bias1/1 -> If Action Subsystem/2(Phase0)
  If Action Subsystem/2(Phase0Event) -> Merge1/2
  If Action Subsystem1/2(Out2) -> Merge1/1
  If Action Subsystem/1(Phi_Out) -> Merge/2
  Add1/1 -> If/2
  Data Type Conversion/1 -> Gain2/1
  Gain3/1 -> Add1/1
  Moving Average1/1 -> Add1/2
  q/1 -> MATLAB Function1/1(u)
  MATLAB Function1/1(y) -> Abs/1
  Abs/1 -> Moving Average1/1, Gain3/1
  Merge1/1 -> Phase0Event/1
  Merge/1 -> Phi_Out/1
  If/2 -> If Action Subsystem/Action
  Add/1 -> If/1
  If/1 -> If Action Subsystem1/Action
  Gain2/1 -> Bias1/1
  Moving Average/1 -> Add/2
  Saturation/1 -> Edge Detector/1
  Edge Detector/1 -> Data Type Conversion/1
  Phi/1 -> If Action Subsystem/1(Phi), Bias2/1
  Bias2/1 -> Saturation/1
  P/1 -> Moving Average/1, Gain1/1
  Gain1/1 -> Add/1
  If Action Subsystem1/1(Out1) -> Merge/1

== system TestStructure/InterForceControlTask/AO2/Subsystem ==
  q : Inport
  f : Inport  Port=2
  Add : Sum  Inputs=++++
  Gain1 : Gain  Gain=1/(2*pi)
  Gain2 : Gain  Gain=1/(2*pi)
  Subsystem : Subsystem
      settings: PortSchema="{\"entries\":[{\"content\":{\"sides\":[{\"content\":{\"connectorIds\":[\"In1\",\"In2\",\"In3\"]},\"type\":\"ConnectorPlacement.EquallySpacedRectSide\",\"uuid\":\"fcadf485-1c54-4f3f-872d-ec2f9b882f19\"},{\"content\":{\"connectorIds\":[\"Out1\",\"Out2\",\"Out3\",\"Out4\"],\"side\":\"RIGHT\"},\"type\":\"ConnectorPlacement.EquallySpacedRectSide\",\"uuid\":\"c1591880-cfe2-422f-a22e-44609bf238b6\"},{\"content\":{\"connectorIds\":[\"In4\"],\"side\":\"TOP\"},\"type\":\"ConnectorPlacement.EquallySpacedRectSide\",\"uuid\":\"5e5eda86-5041-4cab-91db-6a7c0e12be81\"}]},\"type\":\"ConnectorPlacement.EquallySpacedConnector\",\"uuid\":\"19c16159-ed31-430a-9428-452ee8c26aba\"}],\"packageUris\":[\"http://schema.mathworks.com/mf0/Connector/R2020b\"],\"version\":\"1.0\"}"
  Subsystem1 : Subsystem
  Subsystem2 : Subsystem
      settings: PortSchema="{\"entries\":[{\"content\":{\"sides\":[{\"content\":{\"connectorIds\":[\"In1\",\"In2\",\"In3\"]},\"type\":\"ConnectorPlacement.EquallySpacedRectSide\",\"uuid\":\"8ec379b7-ae46-4480-a29c-58696021cca5\"},{\"content\":{\"connectorIds\":[\"Out1\",\"Out2\",\"Out3\"],\"side\":\"RIGHT\"},\"type\":\"ConnectorPlacement.EquallySpacedRectSide\",\"uuid\":\"cda231b2-17f5-4d36-92f5-7ce39ba724b7\"},{\"content\":{\"connectorIds\":[],\"side\":\"TOP\"},\"type\":\"ConnectorPlacement.EquallySpacedRectSide\",\"uuid\":\"4db6421b-b56f-479d-b059-30db4d04c79c\"},{\"content\":{\"connectorIds\":[\"Out4\"],\"side\":\"BOTTOM\"},\"type\":\"ConnectorPlacement.EquallySpacedRectSide\",\"uuid\":\"ff0451e3-8881-4680-9eeb-8c81f572143a\"}]},\"type\":\"ConnectorPlacement.EquallySpacedConnector\",\"uuid\":\"26cfb436-360b-4c37-a6b2-80fa044f0317\"}],\"packageUris\":[\"http://schema.mathworks.com/mf0/Connector/R2020b\"],\"version\":\"1.0\"}"
  Subsystem3 : Subsystem
  Subsystem5 : Subsystem
  x : Outport
  Omega : Outport  Port=2
  Phi : Outport  Port=3
  P : Outport  Port=4
  wires:
  f/1 -> Subsystem/4(f)
  Subsystem/2(Omega) -> Subsystem1/3(Omega), Subsystem3/2(Omega), Subsystem5/3(Omega), Gain1/1
  Subsystem2/4(P) -> P/1
  Subsystem5/1(x) -> Add/4
  Subsystem3/1(x) -> Add/3
  Subsystem2/3(P(t)_Phi) -> Subsystem/3(P(t)_Phi), Subsystem1/2(P(t)_Phi), Subsystem3/3(P(t)_Phi), Subsystem5/2(P(t)_Phi)
  Subsystem1/1(x) -> Add/2
  Subsystem2/2(P(t)_Omega) -> Subsystem/2(P(t)_Omega)
  Subsystem2/1(P(t)_x) -> Subsystem/1(P(t)_x), Subsystem1/1(P(t)_x), Subsystem3/1(P(t)_x), Subsystem5/1(P(t)_x)
  Gain1/1 -> Omega/1
  Subsystem/3(Phi) -> Gain2/1
  Subsystem/1(x) -> Add/1
  Gain2/1 -> Phi/1
  Add/1 -> x/1, Subsystem2/2(X(t))
  q/1 -> Subsystem2/1(T(t))

== system TestStructure/InterForceControlTask/AO2/Subsystem1 ==
  q : Inport
  Math Function : Math  Operator=reciprocal
  Subsystem : Subsystem
  ZeroCrossFinder : Subsystem
  f : Outport
  Peak : Outport  Port=2
  wires:
  Math Function/1 -> f/1
  Subsystem/1(t-t_start) -> Math Function/1
  ZeroCrossFinder/1(Cross) -> Subsystem/1(Peaks), Peak/1
  q/1 -> ZeroCrossFinder/1(q)
